simulink model "DCMotorDisk_sim_2020"  (R2020b)
settings: Solver=ode4  StartTime=0.0  StopTime=10.0  FixedStep=0.05  RelTol=1e-3
settings Model: Creator=005274  LastModifiedBy=005274

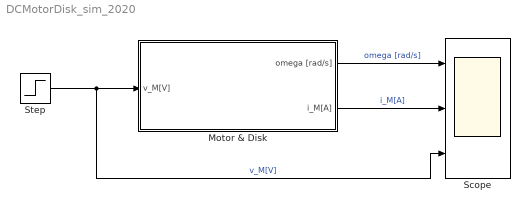
== system DCMotorDisk_sim_2020 ==
  Motor & Disk : Subsystem  mask(DCMotor&DiskModel){R=5.7, L=0.2, J_M=1.1e-4, J_I=1.3e-3, D=6.0e-5, K_tau=7.2e-2, K_e=7.2e-2}
      mask prompts: R "Resistance : R"; L "Inductance : L"; J_M "Moment of Inertia : J_M"; J_I "Moment of Inertia of Load : J_I"; D "Viscus friction : D"; K_tau "Constant torque : K_tau"; K_e "Back electromotive force constant : K_e"
  Scope : Scope  NumInputPorts=3
  Step : Step  After=24  SampleTime=0
  wires:
  Step/1 -> Scope/3, Motor & Disk/1(v_M[V])  "v_M[V]"
  Motor & Disk/1("omega [rad/s] ") -> Scope/1  "omega [rad/s]"
  Motor & Disk/2(i_M[A]) -> Scope/2  "i_M[A]"

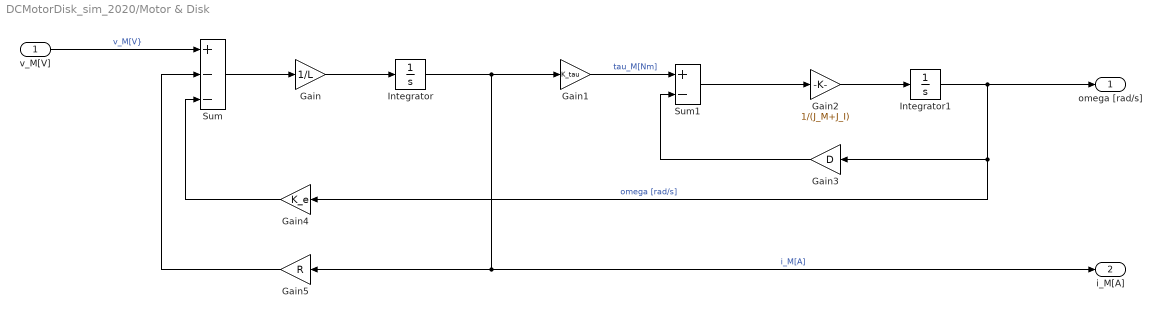
== system DCMotorDisk_sim_2020/Motor & Disk ==
  v_M[V] : Inport
  Gain : Gain  Gain=1/L
  Gain1 : Gain  Gain=K_tau
  Gain2 : Gain  Gain=1/(J_M+J_I)
  Gain3 : Gain  Gain=D
  Gain4 : Gain  Gain=K_e
  Gain5 : Gain  Gain=R
  Integrator : Integrator
  Integrator1 : Integrator
  Sum : Sum  Inputs=+--
  Sum1 : Sum  Inputs=+-
  "omega [rad/s] " : Outport
  i_M[A] : Outport  Port=2
  wires:
  Integrator1/1 -> "omega [rad/s] "/1, Gain4/1, Gain3/1  "omega [rad/s]"
  Sum/1 -> Gain/1
  Gain/1 -> Integrator/1
  Gain5/1 -> Sum/2
  Gain1/1 -> Sum1/1  "tau_M[Nm]"
  Gain2/1 -> Integrator1/1
  Gain3/1 -> Sum1/2
  Gain4/1 -> Sum/3
  Sum1/1 -> Gain2/1
  v_M[V]/1 -> Sum/1  "v_M[V}"
  Integrator/1 -> Gain1/1, Gain5/1, i_M[A]/1  "i_M[A]"
